simulink model "b_microCHP_modulating"  (Simulink 7.6)
settings: Solver=ode45  StartTime=0  StopTime=800000  RelTol=1e-3
model workspace: external: MATLAB File (data not in the file)
undefined symbols (not defined in the file): A, B, C, carmen, Dd, O_th
settings Model: Creator=Sebastian  LastModifiedBy=fabian.ille
settings OptimizationCC: InitFltsAndDblsToZero=on  EfficientMapNaN2IntZero=off
settings DebuggingCC: StrictBusMsg=Warning
settings HardwareCC: TargetIntDivRoundTo=Zero  TargetEndianess=LittleEndian  TargetHWDeviceType=MATLAB Host  ProdEqTarget=off
settings SFSimCC: SimParseCustomCode=off
settings CodeAppCC: MaxIdLength=128

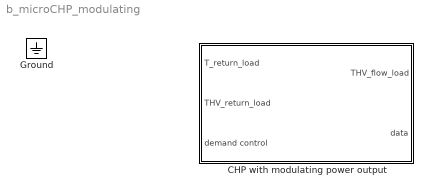
== system b_microCHP_modulating ==
  CHP with modulating power output : Subsystem  mask(CHP ){P_th_max=12500, P_th_min=3500, P_th_start=8000, f_P_el=0.37, T_flow_setpoint=80, T_flow_max=88, t_start=180, t_readjustment=450}
      mask prompts: P_th_max "maximum heating power [W]"; P_th_min "minimum heating power [W]"; P_th_start "initial heating power at start-up phase [W]"; f_P_el "electrical power fraction (referring to heating power) [0..1]"; T_flow_setpoint "flow setpoint temperature [°C]"; T_flow_max "maximum flow temperature [°C]"; t_start "duration of start-up phase [s]"; t_readjustment "duration of readjustment intervall [s]"
      mask help:
      | engine speed = f(T_return_load, T_flow_setpoint, T_flow, T_return)
      | T_return_load: a storage temperature or the return flow temperature.
      | Adjustable start-up phase: initial heating power
      | Ramp-up phase: maximum heating power up to 60°C
      | Control phase: heating power is readjusted after an inputed readjustment intervall.
      |
      | Stateflow needed!
      |
      | Return temperature raising facility.
      mask Help: eval('filetest (''manual.htm#electric_heating'')')
      mask Display: plot(0,0,100,100,[50,50,60,40,50],[55,40,70,60,90],[59,50],[48,40])
  Ground : Ground  IOType=siggen

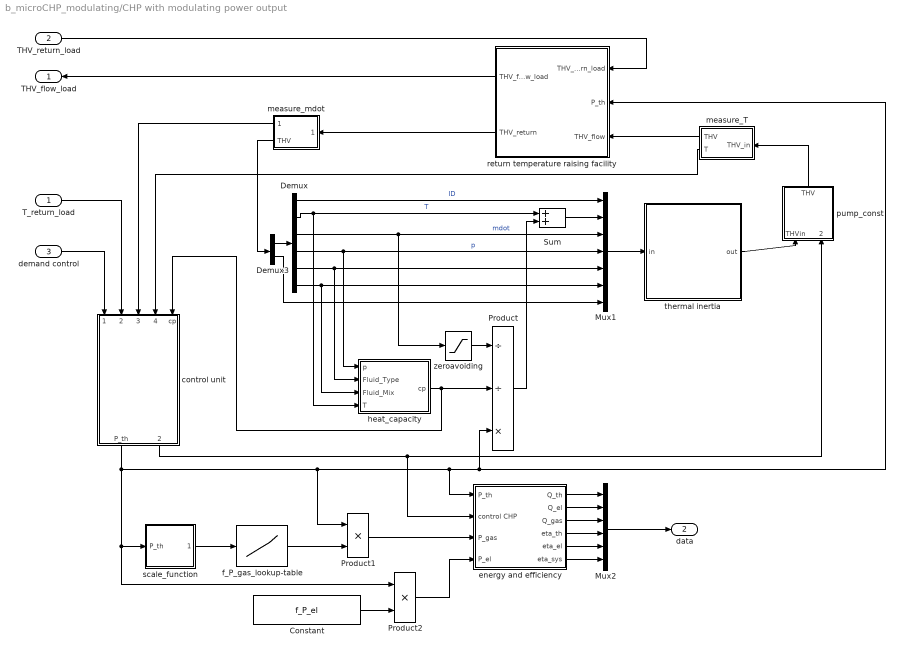
== system b_microCHP_modulating/CHP with modulating power output ==
  T_return_load : Inport
  THV_return_load : Inport  Port=2
  demand control : Inport  Port=3
  Constant : Constant  Value=f_P_el
  Demux : Demux  Outputs=[1 1 1 1 1 1]
  Demux3 : Demux  Outputs=[6 14]
  Mux1 : Mux  Inputs=[1 1 1 1 1 1 14]
  Mux2 : Mux  Inputs=6
  Product : Product  Inputs=//*  SaturateOnIntegerOverflow=on  RndMeth=Zero  InputSameDT=on  OutDataTypeStr=Inherit: Same as first input
  Product1 : Product  Inputs=**  SaturateOnIntegerOverflow=on  RndMeth=Zero  InputSameDT=on  OutDataTypeStr=Inherit: Same as first input
  Product2 : Product  Inputs=**  SaturateOnIntegerOverflow=on  RndMeth=Zero  InputSameDT=on  OutDataTypeStr=Inherit: Same as first input
  Sum : Sum  SaturateOnIntegerOverflow=on  InputSameDT=on  OutDataTypeStr=Inherit: Same as first input
  control unit : Subsystem
      mask Type: control unit
      mask Description:
      | The switching of the CHP depends on the below conditions of safety shutdown and the demand signal of the consumer.
      | conditions of safety shutdown:
      | CHP ON: T_flow < T_flow_max
      | CHP OFF: T_flow > T_flow_max
      mask Display: plot(-30,0,150,100,[70,100,40,10,70,70,10,10],[50,80,80,50,50,20,20,50],[100,70],[50,20],[20,50,50,20,20],[40,40,30,30,40],[62,62,62,61,59,58,58,60],[42,41,39,38,38,40,42,43],[61,62,62,61,60,59,58,58,58,59],[32,31,30,28,27,28,28,30,31,32])
  energy and efficiency : Subsystem
  f_P_gas_lookup-table : Lookup_n-D  NumberOfTableDimensions=1  BreakpointsForDimension1=[1,2]  BreakpointsForDimension2=[44,80]  BreakpointsForDimension3=[1:2]  BreakpointsForDimension4=[1:2]  Table=[1.79 1.5]  InputSameDT=on
  heat_capacity : Subsystem
      mask Type: heat capacity
      mask Description:
      | Calculates the  heat_capacity of fluids [J/(kg*K)].
      | Calls calls the function "hcap" in the CARNOT library "carlib".
      | Definition of the fluid types
      | fluid-ID  material           remarks on fluid mix
      | 1           water              vapourcontent in the 2-phase region
      | 2           air                   is (kg water) / (kg air)
      | 3           cotton oil
      | 4           silicone oil
      | 5           water-glycol    gives the volume partition [0..1] of glycol
      mask Help: eval('htmlhelp (''chap_4_2h.htm#heat_capacity'')')
  measure_T : Subsystem  mask(temperature measurement sensor){tc=10, t0=25}
      mask prompts: tc "time constant of sensor [s]"; t0 "initial temperature [degree centigrade]"
      mask help: Measurement sensor for temperatures with first-oder hold. Temperature is in degree centigrade.
      mask init:
      | tc = 1/max(tc, 0.001);
      mask Help: eval('man (''measure_T'')')
      mask Display: plot(-18,0,30,20,[0 20],[0 0],[10 10 8 8 12 12 10],[0 8 8 17 17 8 8],[10 10 9 9 11 11 10 9],[15 10 10 9 9 10 9 10])
  measure_mdot : Subsystem
      mask Type: massflow measurement sensor
      mask Description: Measurement sensor for massflow in kg/s.
      mask Help: eval('man (''measure_mdot'')')
  pump_const : Subsystem  mask(constant pump){mdotmax=0.3, fluid_id=water, mix=0, dia=0.0157, power=100, p0=3e5}
      mask prompts: mdotmax "massflow rate [kg/s]"; fluid_id "fluid"; mix "percentage of fluid mix [0..1]"; dia "diameter at in- and outlet [m]"; power "electric power consumption [W]"; p0 "system pressure [Pa]"
      mask help: set constant massflow rate
      mask init:
      | mix = min(1, max(0, mix));
      | dia = max(0.001, dia);
      | p0 = max(p0, 1e5);
      mask Help: eval('man(''pump_const'')')
      mask StyleString: edit,popup(water|air|cotton_oil|silicone_oil|water_glycol_mix),edit,edit,edit,edit
      mask Display: plot(0,0,100,100,[40,70,40,30,30,40,60,70,70,60,40],[70,50,30,40,60,70,70,60,40,30,30])
  return temperature raising facility : Subsystem
      mask Type: return temperature raising facility
      mask Description: A return setpoint temperature is calculated depending on heating power and flow setpoint temperature. The thermostatic mixer is located in the return flow of the CHP.
  scale_function : Subsystem
  thermal inertia : Subsystem  LoadFcn=carmen('call');  mask(simple water storage){vol=0.00175*O_th/1000+ 0.0021, d=0.1, stand=standing cylinder, cond=1, uloss=1, tini=25, nodes=3, mpts=1, Tambient=15}
      mask prompts: vol "volume [m³]"; d "diameter [m]"; stand "position"; cond "axial heat conductivity [W/(m*K)]"; uloss "heat loss coefficient [W/(m²*K)]"; tini "initial temperature [degree centigrade]"; nodes "number of nodes"; mpts "number of measurement points (>= 3)  (first is at bottom)"; Tambient "ambient temperature"
      mask help: multinode water storage
      mask init:
      | vol = max(vol, 0.001);
      | d = max(d, 0.001);
      | stand = stand-1;
      | nodes = max(nodes, 1);
      | mpts = max(mpts, 3);
      mask Help: eval('htmlhelp (''chap_4_2s.htm#storage'')')
      mask StyleString: edit,edit,popup(lying cylinder|standing cylinder),edit,edit,edit,edit,edit,edit
      mask Display: plot(0,0,100,110,[40,40,47,53,60,60,53,47,40],[80,40,30,30,40,80,90,90,80],[40,35],[77,77],[64,60],[77,77],[40,35],[42,42],[64,60],[42,42])
  zeroavoiding : Saturate  UpperLimit=inf  LowerLimit=1e-5
  THV_flow_load : Outport  InitialOutput=0
  data : Outport  Port=2  InitialOutput=0
  wires:
  Demux/4 -> Mux1/4, heat_capacity/1(p)  "p"
  Demux/1 -> Mux1/1  "ID"
  Demux/5 -> heat_capacity/2(Fluid_Type), Mux1/5
  Demux/6 -> heat_capacity/3(Fluid_Mix), Mux1/6
  Demux/3 -> Mux1/3, zeroavoiding/1  "mdot"
  Sum/1 -> Mux1/2
  Demux3/1 -> Demux/1
  Demux3/2 -> Mux1/7
  Mux1/1 -> thermal inertia/1(in)
  Product/1 -> Sum/2
  Demux/2 -> heat_capacity/4(T), Sum/1  "T"
  demand control/1 -> control unit/1(demand control)
  T_return_load/1 -> control unit/2(T_return_load)
  heat_capacity/1(cp) -> Product/2, control unit/5(cp)
  measure_T/2(T) -> control unit/4(T_flow)
  measure_mdot/1(mdot) -> control unit/3(mdot_return)
  zeroavoiding/1 -> Product/1
  thermal inertia/1(out) -> pump_const/1(THVin)
  pump_const/1(THV) -> measure_T/1(THV_in)
  control unit/2(control_CHP) -> pump_const/2(control), energy and efficiency/2(control CHP)
  THV_return_load/1 -> return temperature raising facility/1(THV_return_load)
  control unit/1(P_th) -> energy and efficiency/1(P_th), Product/3, return temperature raising facility/2(P_th), Product1/1, scale_function/1(P_th), Product2/1
  scale_function/1(X_pth) -> f_P_gas_lookup-table/1
  Product2/1 -> energy and efficiency/4(P_el)
  f_P_gas_lookup-table/1 -> Product1/2
  Product1/1 -> energy and efficiency/3(P_gas)
  return temperature raising facility/1(THV_flow_load) -> THV_flow_load/1
  return temperature raising facility/2(THV_return) -> measure_mdot/1(THV_in)
  measure_T/1(THV) -> return temperature raising facility/3(THV_flow)
  measure_mdot/2(THV) -> Demux3/1
  Constant/1 -> Product2/2
  energy and efficiency/1(Q_th) -> Mux2/1
  energy and efficiency/2(Q_el) -> Mux2/2
  energy and efficiency/3(Q_gas) -> Mux2/3
  energy and efficiency/4(eta_th) -> Mux2/4
  energy and efficiency/5(eta_el) -> Mux2/5
  energy and efficiency/6(eta_sys) -> Mux2/6
  Mux2/1 -> data/1

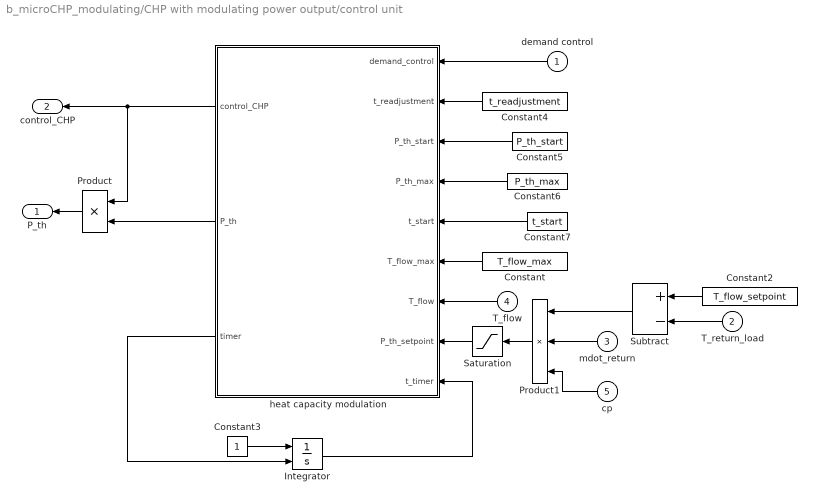
== system b_microCHP_modulating/CHP with modulating power output/control unit ==
  demand control : Inport
  T_return_load : Inport  Port=2
  mdot_return : Inport  Port=3
  T_flow : Inport  Port=4
  cp : Inport  Port=5
  Constant : Constant  Value=T_flow_max
  Constant2 : Constant  Value=T_flow_setpoint
  Constant3 : Constant
  Constant4 : Constant  Value=t_readjustment
  Constant5 : Constant  Value=P_th_start
  Constant6 : Constant  Value=P_th_max
  Constant7 : Constant  Value=t_start
  Integrator : Integrator  ExternalReset=rising
  Product : Product  Inputs=**  SaturateOnIntegerOverflow=on  RndMeth=Zero  InputSameDT=on  OutDataTypeStr=Inherit: Same as first input
  Product1 : Product  Inputs=***  SaturateOnIntegerOverflow=on  RndMeth=Zero  InputSameDT=on  OutDataTypeStr=Inherit: Same as first input
  Saturation : Saturate  UpperLimit=P_th_max  LowerLimit=P_th_min
  Subtract : Sum  Inputs=+-
  heat capacity modulation : Stateflow chart  TreatAsAtomicUnit=on
  P_th : Outport
  control_CHP : Outport  Port=2
  wires:
  heat capacity modulation/3(timer) -> Integrator/2
  Constant/1 -> heat capacity modulation/6(T_flow_max)
  Constant3/1 -> Integrator/1
  Constant4/1 -> heat capacity modulation/2(t_readjustment)
  mdot_return/1 -> Product1/2
  cp/1 -> Product1/3
  Constant5/1 -> heat capacity modulation/3(P_th_start)
  Constant6/1 -> heat capacity modulation/4(P_th_max)
  Constant7/1 -> heat capacity modulation/5(t_start)
  Constant2/1 -> Subtract/1
  demand control/1 -> heat capacity modulation/1(demand_control)
  Subtract/1 -> Product1/1
  T_flow/1 -> heat capacity modulation/7(T_flow)
  T_return_load/1 -> Subtract/2
  Product/1 -> P_th/1
  Product1/1 -> Saturation/1
  Saturation/1 -> heat capacity modulation/8(P_th_setpoint)
  heat capacity modulation/1(control_CHP) -> control_CHP/1, Product/1
  Integrator/1 -> heat capacity modulation/9(t_timer)
  heat capacity modulation/2(P_th) -> Product/2

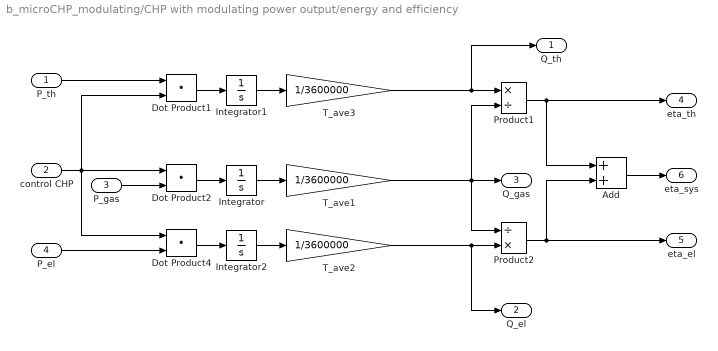
== system b_microCHP_modulating/CHP with modulating power output/energy and efficiency ==
  P_th : Inport
  control CHP : Inport  Port=2
  P_gas : Inport  Port=3
  P_el : Inport  Port=4
  Add : Sum
  Dot Product1 : DotProduct  InputSameDT=on  OutDataTypeStr=Inherit: Inherit via internal rule
  Dot Product2 : DotProduct  InputSameDT=on  OutDataTypeStr=Inherit: Inherit via internal rule
  Dot Product4 : DotProduct  InputSameDT=on  OutDataTypeStr=Inherit: Inherit via internal rule
  Integrator : Integrator
  Integrator1 : Integrator
  Integrator2 : Integrator
  Product1 : Product  Inputs=*/  SaturateOnIntegerOverflow=on  RndMeth=Zero  InputSameDT=on  OutDataTypeStr=Inherit: Same as first input
  Product2 : Product  Inputs=/*  SaturateOnIntegerOverflow=on  RndMeth=Zero  InputSameDT=on  OutDataTypeStr=Inherit: Same as first input
  T_ave1 : Gain  Gain=1/3600000  SaturateOnIntegerOverflow=on  OutDataTypeStr=Inherit: Same as input  ParamDataTypeStr=Inherit: Same as input
  T_ave2 : Gain  Gain=1/3600000  SaturateOnIntegerOverflow=on  OutDataTypeStr=Inherit: Same as input  ParamDataTypeStr=Inherit: Same as input
  T_ave3 : Gain  Gain=1/3600000  SaturateOnIntegerOverflow=on  OutDataTypeStr=Inherit: Same as input  ParamDataTypeStr=Inherit: Same as input
  Q_th : Outport  InitialOutput=0
  Q_el : Outport  Port=2  InitialOutput=0
  Q_gas : Outport  Port=3  InitialOutput=0
  eta_th : Outport  Port=4  InitialOutput=0
  eta_el : Outport  Port=5  InitialOutput=0
  eta_sys : Outport  Port=6  InitialOutput=0
  wires:
  P_gas/1 -> Dot Product2/2
  Integrator/1 -> T_ave1/1
  Integrator2/1 -> T_ave2/1
  P_el/1 -> Dot Product4/2
  Product2/1 -> eta_el/1, Add/2
  Dot Product4/1 -> Integrator2/1
  Dot Product2/1 -> Integrator/1
  control CHP/1 -> Dot Product2/1, Dot Product4/1, Dot Product1/2
  T_ave1/1 -> Product2/1, Q_gas/1, Product1/2
  T_ave2/1 -> Product2/2, Q_el/1
  Dot Product1/1 -> Integrator1/1
  P_th/1 -> Dot Product1/1
  Integrator1/1 -> T_ave3/1
  T_ave3/1 -> Product1/1, Q_th/1
  Product1/1 -> Add/1, eta_th/1
  Add/1 -> eta_sys/1

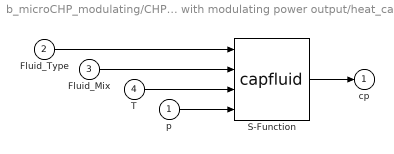
== system b_microCHP_modulating/CHP with modulating power output/heat_capacity ==
  p : Inport
  Fluid_Type : Inport  Port=2
  Fluid_Mix : Inport  Port=3
  T : Inport  Port=4
  S-Function : S-Function  FunctionName=capfluid  EnableBusSupport=off
      mask Description:
      | Calculates the heat_capacity
      | 
      | INPUT VECTORS:
      | fluid type [1..5]
      | fluid mix
      | temperature [°C]
      | pressure [Pa]
      | 
      | OUTPUT VECTOR:
      | heat_capacity [J/(kg K)]
  cp : Outport  InitialOutput=0
  wires:
  p/1 -> S-Function/4
  T/1 -> S-Function/3
  Fluid_Mix/1 -> S-Function/2
  Fluid_Type/1 -> S-Function/1
  S-Function/1 -> cp/1

== system b_microCHP_modulating/CHP with modulating power output/measure_T ==
  THV_in : Inport
  heat capacity : StateSpace  A=-tc  B=tc  D=0  X0=t0
  select temperature : Selector  InputPortWidth=20  IndexOptions=Index vector (dialog)  Indices=[2]  OutputSizes=1
  THV : Outport  InitialOutput=0
  T : Outport  Port=2  InitialOutput=0
  wires:
  THV_in/1 -> select temperature/1, THV/1
  select temperature/1 -> heat capacity/1
  heat capacity/1 -> T/1

== system b_microCHP_modulating/CHP with modulating power output/measure_mdot ==
  THV_in : Inport
  select massflow : Selector  InputPortWidth=20  IndexOptions=Index vector (dialog)  Indices=[3]  OutputSizes=1
  mdot : Outport  InitialOutput=0
  THV : Outport  Port=2  InitialOutput=0
  wires:
  THV_in/1 -> select massflow/1, THV/1
  select massflow/1 -> mdot/1

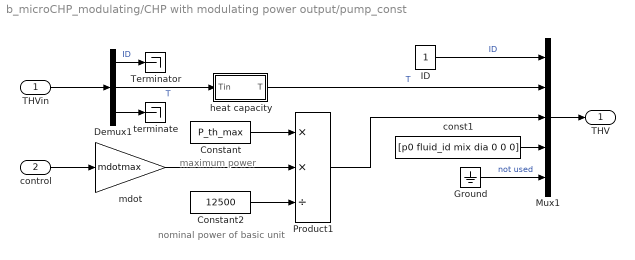
== system b_microCHP_modulating/CHP with modulating power output/pump_const ==
  note: maximum power
  note: nominal power of basic unit
  THVin : Inport
  control : Inport  Port=2
  Constant : Constant  Value=P_th_max
  Constant2 : Constant  Value=12500
  Demux1 : Demux  Outputs=[1 1 18]
  Ground : Ground
  ID : Constant
  Mux1 : Mux  Inputs=[1 1 1 7 10]
  Product1 : Product  Inputs=**/  SaturateOnIntegerOverflow=on  RndMeth=Zero  InputSameDT=on  OutDataTypeStr=Inherit: Same as first input
  Terminator : Terminator
  const1 : Constant  Value=[p0 fluid_id mix dia 0 0 0]
  heat capacity : Subsystem  mask{NTU=3.1}
      mask prompts: NTU "NTU (k*A/(m*cp))"
  mdot : Gain  Gain=mdotmax  SaturateOnIntegerOverflow=on  OutDataTypeStr=Inherit: Same as input  ParamDataTypeStr=Inherit: Same as input
  terminate : Terminator
  THV : Outport  InitialOutput=0
  wires:
  Ground/1 -> Mux1/5  "not used"
  Demux1/3 -> terminate/1
  THVin/1 -> Demux1/1
  ID/1 -> Mux1/1  "ID"
  Mux1/1 -> THV/1
  const1/1 -> Mux1/4
  Demux1/1 -> Terminator/1  "ID"
  Demux1/2 -> heat capacity/1(Tin)  "T"
  mdot/1 -> Product1/2
  Constant/1 -> Product1/1
  Constant2/1 -> Product1/3
  Product1/1 -> Mux1/3
  heat capacity/1(T) -> Mux1/2  "T"
  control/1 -> mdot/1

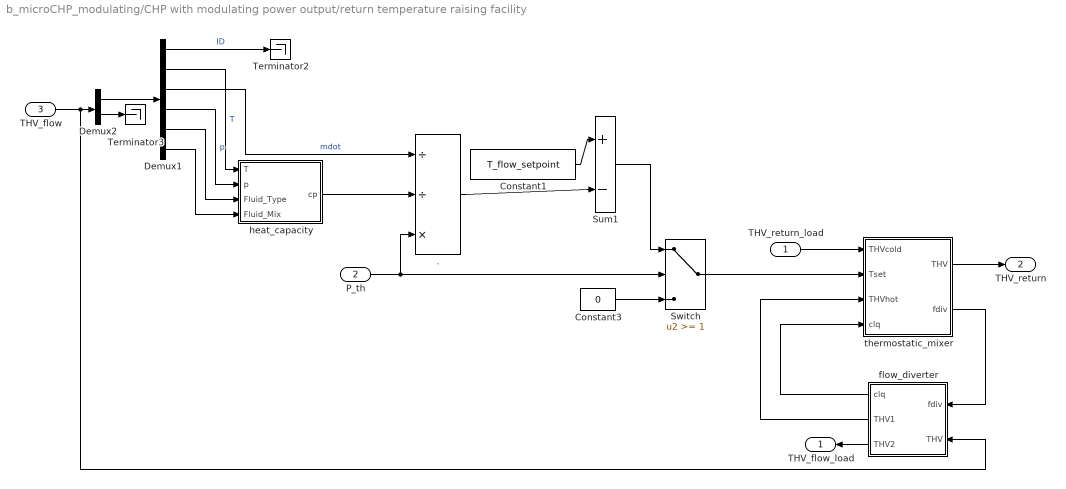
== system b_microCHP_modulating/CHP with modulating power output/return temperature raising facility ==
  THV_return_load : Inport
  P_th : Inport  Port=2
  THV_flow : Inport  Port=3
  . : Product  Inputs=//*  SaturateOnIntegerOverflow=on  RndMeth=Zero  InputSameDT=on  OutDataTypeStr=Inherit: Same as first input
  Constant1 : Constant  Value=T_flow_setpoint
  Constant3 : Constant  Value=0
  Demux1 : Demux  Outputs=[1 1 1 1 1 1]
  Demux2 : Demux  Outputs=[6 -1]
  Sum1 : Sum  Inputs=|+-  SaturateOnIntegerOverflow=on  InputSameDT=on  OutDataTypeStr=Inherit: Same as first input
  Switch : Switch  Threshold=1  SaturateOnIntegerOverflow=on  InputSameDT=on
  Terminator2 : Terminator
  Terminator3 : Terminator
  flow_diverter : Subsystem  mask(flow diverter, fixed rate){t=1}
      mask prompts: t "time constant in s"
      mask help:
      | The block diverts an incoming massflow according to:
      | mdot1 = mdot * fdiv
      | mdot2 = mdot * (1-fdiv)
      | fdiv is limited to the range [0..1]
      mask init:
      | t = max(0.001, t);
      mask Help: eval('man(''flow_diverter_fixed_rate'')')
      mask Display: plot(0,-5,120,65,[20 45 20 20],[20 30 40 20],[45 70 70 45],[30 20 40 30],[45 35 55 45],[30 10 10 30])
  heat_capacity : Subsystem
      mask Type: heat capacity
      mask Description:
      | Calculates the  heat_capacity of fluids [J/(kg*K)].
      | Calls calls the function "hcap" in the CARNOT library "carlib".
      | Definition of the fluid types
      | fluid-ID  material           remarks on fluid mix
      | 1           water              vapourcontent in the 2-phase region
      | 2           air                   is (kg water) / (kg air)
      | 3           cotton oil
      | 4           silicone oil
      | 5           water-glycol    gives the volume partition [0..1] of glycol
      | 6           tyfocor LS      only available in liquid phase
      mask Help: eval('man(''heat_capacity'')')
  thermostatic_mixer : Subsystem  mask(thermostatic flow mixer){t=1}
      mask prompts: t "time constant for valve [s]"
      mask help:
      | The thermostatic flow mixer mixes cold and hot fluid to set a desired temperature and calculates the pressure drop.
      | Use together with flow_diverter_fixed_rate.
      mask init:
      | t = max(t, 0.01);
      | t1 = 1/t;
      mask Help: eval('man(''flow_mixer_thermostatic'')')
      mask Display: plot(-10,0,90,100,[40,60,60,40,40],[60,40,60,40,60],[44,50,56,44],[66,50,66,66],[50,50],[30,50],[56,44],[25,25],[50,50],[10,25])
  THV_flow_load : Outport
  THV_return : Outport  Port=2
  wires:
  Demux1/1 -> Terminator2/1  "ID"
  P_th/1 -> ./3, Switch/2
  heat_capacity/1(cp) -> ./2
  THV_flow/1 -> Demux2/1, flow_diverter/2(THV)
  Demux2/1 -> Demux1/1
  Demux1/2 -> heat_capacity/1(T)  "T"
  Demux1/3 -> ./1  "mdot"
  Demux1/6 -> heat_capacity/4(Fluid_Mix)
  Demux1/5 -> heat_capacity/3(Fluid_Type)
  Demux1/4 -> heat_capacity/2(p)  "p"
  flow_diverter/1(clq) -> thermostatic_mixer/4(clq)
  flow_diverter/3(THV2) -> THV_flow_load/1
  THV_return_load/1 -> thermostatic_mixer/1(THVcold)
  flow_diverter/2(THV1) -> thermostatic_mixer/3(THVhot)
  thermostatic_mixer/2(fdiv) -> flow_diverter/1(fdiv)
  Demux2/2 -> Terminator3/1
  Constant1/1 -> Sum1/1
  Sum1/1 -> Switch/1
  ./1 -> Sum1/2
  Constant3/1 -> Switch/3
  Switch/1 -> thermostatic_mixer/2(Tset)
  thermostatic_mixer/1(THV) -> THV_return/1

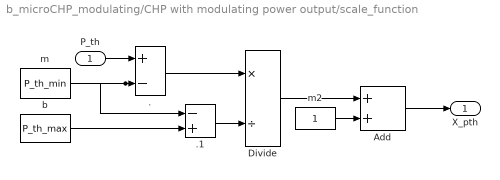
== system b_microCHP_modulating/CHP with modulating power output/scale_function ==
  P_th : Inport
  . : Sum  Inputs=+-
  .1 : Sum  Inputs=-+
  Add : Sum
  Divide : Product  Inputs=*/
  b : Constant  Value=P_th_max
  m : Constant  Value=P_th_min
  m2 : Constant
  X_pth : Outport  InitialOutput=0
  wires:
  m2/1 -> Add/2
  m/1 -> ./2, .1/1
  ./1 -> Divide/1
  b/1 -> .1/2
  .1/1 -> Divide/2
  P_th/1 -> ./1
  Divide/1 -> Add/1
  Add/1 -> X_pth/1

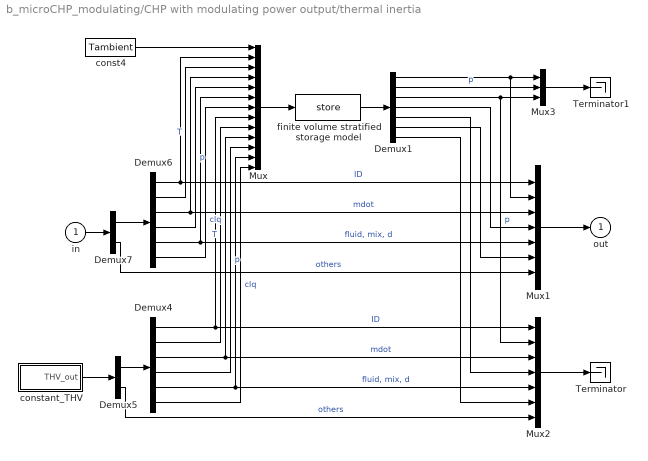
== system b_microCHP_modulating/CHP with modulating power output/thermal inertia ==
  in : Inport
  Demux1 : Demux  Outputs=[1 mpts-2 1 1 1 3 3]
  Demux4 : Demux  Outputs=[1 1 1 1 3 3]
  Demux5 : Demux  Outputs=[10 -1]
  Demux6 : Demux  Outputs=[1 1 1 1 3 3]
  Demux7 : Demux  Outputs=[10 -1]
  Mux : Mux  Inputs=13
  Mux1 : Mux  Inputs=7
  Mux2 : Mux  Inputs=7
  Mux3 : Mux  Inputs=3
  Terminator : Terminator
  Terminator1 : Terminator
  const4 : Constant  Value=Tambient
  constant_THV : Subsystem  mask(constant THV){t=20, mdot=0, p=2e5, fluid=water, mix=0, dia=0.02}
      mask prompts: t "temperature [degree centigrade]"; mdot "massflow [kg/s]"; p "pressure [Pa]"; mix "fluid mixture [0..1]"; dia "diameter [m]"
      mask help: Create a constant Thermo-Hydraulic-Vector.
      mask init:
      | mix = min(1, max(0, mix));
      | dia = max(dia, 0.001);
      mask Help: eval('man (''constant_THV'')')
      mask StyleString: edit,edit,edit,popup(water|air|cotton_oil|silicone_oil|water_glycol_mix|tyfocor_LS),edit,edit
  finite volume stratified storage model : S-Function  FunctionName=store  Parameters=vol, d, stand, uloss, cond, tini, nodes, mpts  EnableBusSupport=off
  out : Outport  InitialOutput=0
  wires:
  Demux1/7 -> Mux2/6
  Demux5/2 -> Mux2/7  "others"
  Demux1/6 -> Mux1/6
  Demux1/5 -> Mux2/4
  Demux4/2 -> Mux/9  "T"
  Mux2/1 -> Terminator/1
  Demux4/4 -> Mux/11  "p"
  Demux4/6 -> Mux/13  "clq"
  Demux5/1 -> Demux4/1
  Demux4/1 -> Mux/8, Mux2/1  "ID"
  Demux4/3 -> Mux/10, Mux2/3  "mdot"
  Demux4/5 -> Mux/12, Mux2/5  "fluid, mix, d"
  constant_THV/1(THV_out) -> Demux5/1
  Demux7/2 -> Mux1/7  "others"
  Demux1/3 -> Mux3/3, Mux2/2  "p"
  Demux1/2 -> Mux3/2  "p"
  Demux1/1 -> Mux3/1, Mux1/2
  Mux3/1 -> Terminator1/1
  Demux6/6 -> Mux/7  "clq"
  Demux7/1 -> Demux6/1
  in/1 -> Demux7/1
  Demux1/4 -> Mux1/4
  Mux/1 -> finite volume stratified storage model/1
  const4/1 -> Mux/1
  Mux1/1 -> out/1
  Demux6/1 -> Mux1/1, Mux/2  "ID"
  Demux6/2 -> Mux/3  "T"
  Demux6/3 -> Mux/4, Mux1/3  "mdot"
  Demux6/4 -> Mux/5  "p"
  finite volume stratified storage model/1 -> Demux1/1
  Demux6/5 -> Mux/6, Mux1/5  "fluid, mix, d"

== system b_microCHP_modulating/CHP with modulating power output/pump_const/heat capacity ==
  Tin : Inport
  heat capacity : StateSpace  A=-NTU  B=NTU  D=0  X0=80
  T : Outport
  wires:
  heat capacity/1 -> T/1
  Tin/1 -> heat capacity/1

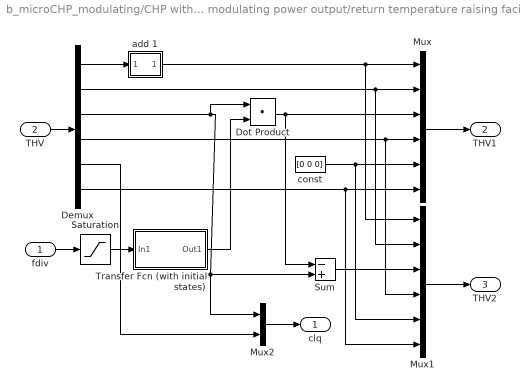
== system b_microCHP_modulating/CHP with modulating power output/return temperature raising facility/flow_diverter ==
  fdiv : Inport
  THV : Inport  Port=2
  Demux : Demux  Outputs=[1 1 1 4 3 10]
  Dot Product : DotProduct  InputSameDT=on  OutDataTypeStr=Inherit: Inherit via internal rule
  Mux : Mux  Inputs=6
  Mux1 : Mux  Inputs=6
  Mux2 : Mux  Inputs=2
  Saturation : Saturate  UpperLimit=1  LowerLimit=0
  Sum : Sum  Inputs=-+  SaturateOnIntegerOverflow=on  InputSameDT=on  OutDataTypeStr=Inherit: Same as first input
  Transfer Fcn (with initial states) : Subsystem  mask(Transfer Function with Initial States){N=[1], D=[t  1], X0=.5}
      mask prompts: N "Numerator:"; D "Denominator:"; X0 "Initial conditions:"
      mask help: Vector expressions for numerator, and denominator. Coefficients are in descending powers of s.
      mask init:
      | [A,B,C,Dd]=tf2ss(N,D);if (isempty(X0));[m,n]=size(A);X0=zeros(1,m); end;
      mask Help: Specify the initial states for the transfer function.  The state ordering is determined by the m-file tf2ss.  There is no unique mapping of the states in a transfer function to states in a state-space representation.  However, tf2ss will consistently use the same mapping for a given transfer function.
      mask Display: dpoly(N,D,'s')
  add 1 : Subsystem  mask(add constant){c=1}
      mask prompts: c "constant c"
      mask help: This block adds a constant c to each element of the input vector.
      mask Help: eval('man (''add_constant'')')
      mask Display: disp('+c');
  const : Constant  Value=[0 0 0]
  clq : Outport  InitialOutput=0
  THV1 : Outport  Port=2  InitialOutput=0
  THV2 : Outport  Port=3  InitialOutput=0
  wires:
  Dot Product/1 -> Mux/3, Sum/1
  fdiv/1 -> Saturation/1
  Saturation/1 -> Transfer Fcn (with initial states)/1(In1)
  Demux/6 -> Mux/6, Mux1/6
  THV/1 -> Demux/1
  Mux1/1 -> THV2/1
  Mux/1 -> THV1/1
  Demux/4 -> Mux/4, Mux1/4
  const/1 -> Mux/5, Mux1/5
  Demux/5 -> Mux2/2
  Demux/3 -> Sum/2, Mux2/1, Dot Product/1
  Sum/1 -> Mux1/3
  Mux2/1 -> clq/1
  Demux/2 -> Mux/2, Mux1/2
  Transfer Fcn (with initial states)/1(Out1) -> Dot Product/2
  Demux/1 -> add 1/1(In1)
  add 1/1(Out1) -> Mux/1, Mux1/1

== system b_microCHP_modulating/CHP with modulating power output/return temperature raising facility/heat_capacity ==
  T : Inport
  p : Inport  Port=2
  Fluid_Type : Inport  Port=3
  Fluid_Mix : Inport  Port=4
  S-Function : S-Function  FunctionName=capfluid  EnableBusSupport=off
  cp : Outport  InitialOutput=0
  wires:
  S-Function/1 -> cp/1
  Fluid_Type/1 -> S-Function/1
  Fluid_Mix/1 -> S-Function/2
  T/1 -> S-Function/3
  p/1 -> S-Function/4

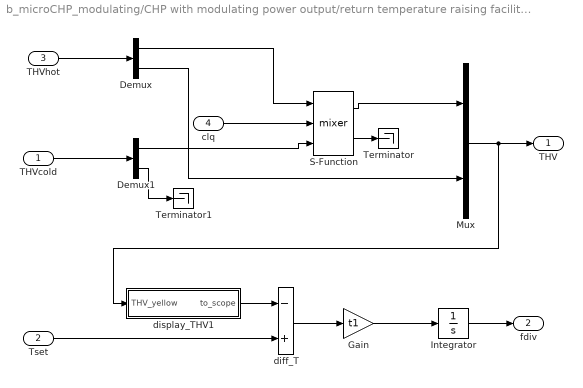
== system b_microCHP_modulating/CHP with modulating power output/return temperature raising facility/thermostatic_mixer ==
  THVcold : Inport
  Tset : Inport  Port=2
  THVhot : Inport  Port=3
  clq : Inport  Port=4
  Demux : Demux  Outputs=[10 10]
  Demux1 : Demux  Outputs=[10 10]
  Gain : Gain  Gain=t1  SaturateOnIntegerOverflow=on  OutDataTypeStr=Inherit: Same as input  ParamDataTypeStr=Inherit: Same as input
  Integrator : Integrator  LimitOutput=on  UpperSaturationLimit=1  LowerSaturationLimit=0
  Mux : Mux  Inputs=2
  S-Function : S-Function  FunctionName=mixer  Parameters=t1  EnableBusSupport=off
  Terminator : Terminator
  Terminator1 : Terminator
  diff_T : Sum  Inputs=-+  SaturateOnIntegerOverflow=on  InputSameDT=on  OutDataTypeStr=Inherit: Same as first input
  display_THV1 : Subsystem  mask(display from THV){t=on, m=off, p=off, id=off, mix=off, d=off}
      mask prompts: t "temperature [degree centigrade]"; m "massflow [kg/s]"; p "pressure [Pa]"; id "fluid ID (1 = water, 2 = air, 3 = cotton oil, 4 = water-glycol)"; mix "fluid mix"; d "diameter [m]"
      mask help: Displays the ticked values from one THV
      mask init:
      | v=[];
      | if (t)
      |     v  = [2];
      | end
      | if (m)
      |     v= [v 3];
      | end
      | if (p)
      |     v = [v 4];
      | end
      | if (id)
      |     v = [v 5];
      | end
      | if (mix)
      |     v = [v 6];
      | end
      | if (d)
      |     v = [v 7];
      | end
      mask Help: eval('man(''display_THV'')')
  THV : Outport  InitialOutput=0
  fdiv : Outport  Port=2  InitialOutput=0
  wires:
  Mux/1 -> THV/1, display_THV1/1(THV_yellow)
  Demux/1 -> S-Function/1
  THVcold/1 -> Demux1/1
  THVhot/1 -> Demux/1
  Tset/1 -> diff_T/2
  display_THV1/1(to_scope) -> diff_T/1
  diff_T/1 -> Gain/1
  S-Function/1 -> Mux/1
  clq/1 -> S-Function/2
  Demux1/1 -> S-Function/3
  S-Function/2 -> Terminator/1
  Gain/1 -> Integrator/1
  Demux1/2 -> Terminator1/1
  Demux/2 -> Mux/2
  Integrator/1 -> fdiv/1

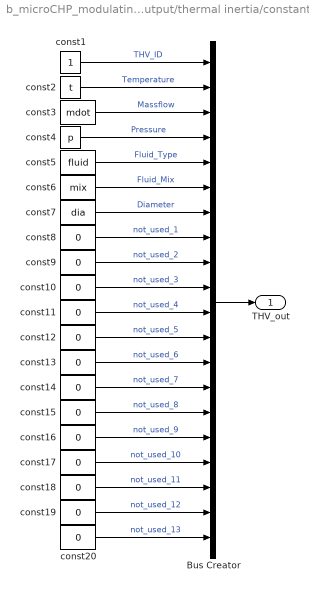
== system b_microCHP_modulating/CHP with modulating power output/thermal inertia/constant_THV ==
  Bus Creator : BusCreator  Inputs=20
  const1 : Constant
  const{8..20} (13 alike) : Constant  Value=0
  const2 : Constant  Value=t
  const3 : Constant  Value=mdot
  const4 : Constant  Value=p
  const5 : Constant  Value=fluid
  const6 : Constant  Value=mix
  const7 : Constant  Value=dia
  THV_out : Outport  InitialOutput=0
  wires:
  const20/1 -> Bus Creator/20  "not_used_13"
  const19/1 -> Bus Creator/19  "not_used_12"
  const18/1 -> Bus Creator/18  "not_used_11"
  const17/1 -> Bus Creator/17  "not_used_10"
  const16/1 -> Bus Creator/16  "not_used_9"
  const15/1 -> Bus Creator/15  "not_used_8"
  const14/1 -> Bus Creator/14  "not_used_7"
  const13/1 -> Bus Creator/13  "not_used_6"
  const12/1 -> Bus Creator/12  "not_used_5"
  const11/1 -> Bus Creator/11  "not_used_4"
  const10/1 -> Bus Creator/10  "not_used_3"
  const9/1 -> Bus Creator/9  "not_used_2"
  const8/1 -> Bus Creator/8  "not_used_1"
  const7/1 -> Bus Creator/7  "Diameter"
  const6/1 -> Bus Creator/6  "Fluid_Mix"
  const5/1 -> Bus Creator/5  "Fluid_Type"
  const4/1 -> Bus Creator/4  "Pressure"
  const3/1 -> Bus Creator/3  "Massflow"
  const2/1 -> Bus Creator/2  "Temperature"
  const1/1 -> Bus Creator/1  "THV_ID"
  Bus Creator/1 -> THV_out/1

== system b_microCHP_modulating/CHP with modulating power output/return temperature raising facility/flow_diverter/Transfer Fcn (with initial states) ==
  In1 : Inport
  State Space : StateSpace  A=A  B=B  C=C  D=Dd  X0=X0
  Out1 : Outport  InitialOutput=0
  wires:
  State Space/1 -> Out1/1
  In1/1 -> State Space/1

== system b_microCHP_modulating/CHP with modulating power output/return temperature raising facility/flow_diverter/add 1 ==
  In1 : Inport
  Sum : Sum  SaturateOnIntegerOverflow=on  InputSameDT=on  OutDataTypeStr=Inherit: Same as first input
  const : Constant  Value=c
  Out1 : Outport  InitialOutput=0
  wires:
  Sum/1 -> Out1/1
  In1/1 -> Sum/2
  const/1 -> Sum/1

== system b_microCHP_modulating/CHP with modulating power output/return temperature raising facility/thermostatic_mixer/display_THV1 ==
  THV_yellow : Inport
  Selector : Selector  InputPortWidth=20  IndexOptions=Index vector (dialog)  Indices=[v]  OutputSizes=1
  to_scope : Outport  InitialOutput=0
  wires:
  Selector/1 -> to_scope/1
  THV_yellow/1 -> Selector/1

== stateflow chart CHP with modulating power output/control unit/heat capacity modulation ==
  state OFF/
    entry:control_CHP=0;
    timer=0;
  state P_th_modulation
    state control_phase/
      entry:
      timer=0;
      P_th=P_th_setpoint;
    state ramp_up_phase/
      entry: P_th=P_th_max;
    state start_up_phase/
      entry:control_CHP=1;
      timer=1;
      P_th=P_th_start;
    state readjustment_intervall/
      entry:
      timer=1;
    control_phase -> readjustment_intervall
    (default) -> start_up_phase
    readjustment_intervall -> control_phase : [t_timer>t_readjustment]
    start_up_phase -> ramp_up_phase : [t_timer>t_start]
    ramp_up_phase -> control_phase : [T_flow>60]
  (default) -> OFF
  OFF -> P_th_modulation : [ T_flow<T_flow_max & demand_control==1]
  P_th_modulation -> OFF : [T_flow>T_flow_max | demand_control==0]
  data: demand_control input double; t_readjustment input double; P_th_start input double; P_th_max input double; t_start input double; T_flow_max input double; control_CHP output double; T_flow input double; P_th output double =2050; timer output double; P_th_setpoint input double; t_timer input double
